simulink model "Lab4_GaussianFilter"  (Simulink 10.2)
settings: Solver=VariableStepAuto  StartTime=0.0  StopTime=10  RelTol=1e-3
libraries: commrandsrc3 x1, commutil2 x1
settings Model: Creator=Newtr  LastModifiedBy=Newtr
settings DataIOCC: SaveFormat=Dataset  SignalLoggingSaveFormat=Dataset  ReturnWorkspaceOutputs=on
settings OptimizationCC: LifeSpan=auto
settings DebuggingCC: UnderspecifiedInitializationDetection=Simplified  MergeDetectMultiDrivingBlocksExec=error  FcnCallInpInsideContextMsg=error  SFUnexpectedBacktrackingDiag=error  SFNoUnconditionalDefaultTransitionDiag=error  SFExecutionAtInitializationDiag=warning  ArithmeticOperatorsInVariantConditions=error
settings HardwareCC: ProdBitPerPointer=64  ProdBitPerSizeT=64  ProdBitPerPtrDiffT=64  ProdLargestAtomicFloat=Float  ProdIntDivRoundTo=Zero  ProdEndianess=LittleEndian  ProdWordSize=64  ProdHWDeviceType=Intel->x86-64 (Windows64)
settings ModelReferenceCC: PropagateSignalLabelsOutOfModel=on
settings SFSimCC: SimUseLocalCustomCode=on  CustomCodeUndefinedFunction=FilterOut
settings RTWCC: RTWUseLocalCustomCode=on
settings CodeAppCC: StateflowObjectComments=off
settings GRTTargetCC: TargetLangStandard=C99 (ISO)  CombineOutputUpdateFcns=on  GRTInterface=off
settings ConfigComp: CovMetricSettings=dwe  CovSaveCumulativeToWorkspaceVar=off  CovSaveSingleToWorkspaceVar=off  CovExternalEMLEnable=on

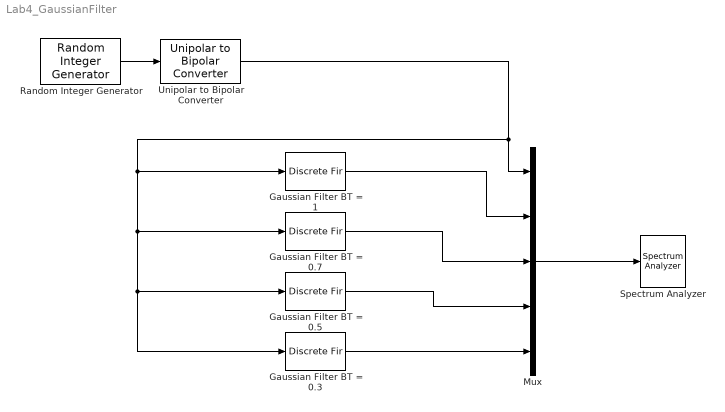
== system Lab4_GaussianFilter ==
  Gaussian Filter BT = 0.3 : DiscreteFir  Coefficients=0.3
  Gaussian Filter BT = 0.5 : DiscreteFir  Coefficients=0.5
  Gaussian Filter BT = 0.7 : DiscreteFir  Coefficients=0.7
  Gaussian Filter BT = 1 : DiscreteFir  Coefficients=1
  Mux : Mux  Inputs=5
  Random Integer Generator : commrandsrc3/Random Integer Generator  SetSize=2  SeedSource=Parameter  Seed=500  SampleTime=1/270000  SamplesPerFrame=1  OutputDataType=double  SimulateUsing=Interpreted execution
  Spectrum Analyzer : SpectrumAnalyzer
  Unipolar to Bipolar Converter : commutil2/Unipolar to Bipolar Converter  M=2  polarity=Positive  dataType=Inherit via internal rule
  wires:
  Random Integer Generator/1 -> Unipolar to Bipolar Converter/1
  Gaussian Filter BT = 0.3/1 -> Mux/5
  Gaussian Filter BT = 0.5/1 -> Mux/4
  Gaussian Filter BT = 0.7/1 -> Mux/3
  Gaussian Filter BT = 1/1 -> Mux/2
  Unipolar to Bipolar Converter/1 -> Gaussian Filter BT = 1/1, Gaussian Filter BT = 0.7/1, Gaussian Filter BT = 0.5/1, Gaussian Filter BT = 0.3/1, Mux/1
  Mux/1 -> Spectrum Analyzer/1
